simulink library "SUB_L4_Task_10ms_SUB_BRKPEDARB"  (R2018a)
settings: Solver=VariableStepAuto  StartTime=0.0  StopTime=10.0  RelTol=1e-3
libraries: EmE_MBD_Blockset x73, PTC_MBDS_LIB x6, simulink x3
(part 1 of 2)
settings Model: Creator=Chris.Balton  LastModifiedBy=Gavin.Coelho

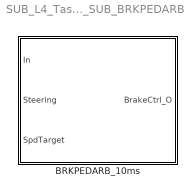
== system SUB_L4_Task_10ms_SUB_BRKPEDARB ==
  BRKPEDARB_10ms : Subsystem

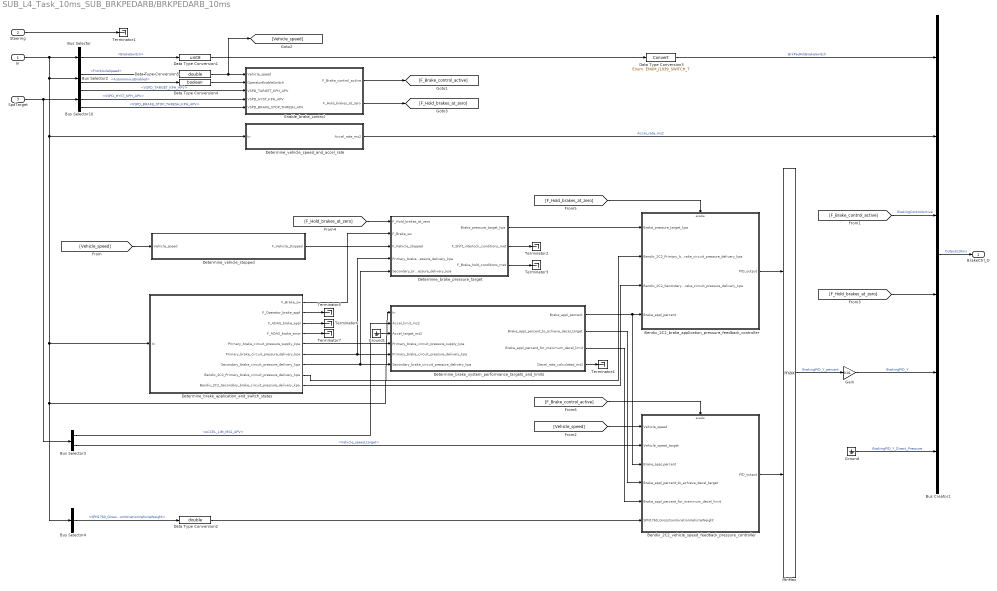
== system SUB_L4_Task_10ms_SUB_BRKPEDARB/BRKPEDARB_10ms ==
  In : Inport
  Steering : Inport  Port=2
  SpdTarget : Inport  Port=3
  Bendix_2C2_brake_application_pressure_feedback_controller : Subsystem  TreatAsAtomicUnit=on
  Bendix_2C2_vehicle_speed_feedback_pressure_controller : Subsystem  TreatAsAtomicUnit=on
  Bus Creator1 : BusCreator  Inputs=6
  Bus Selector : BusSelector  OutputSignals=CAN.CCVS_31.BrakeSwitch
  Bus Selector10 : BusSelector  OutputSignals=VSPD_TARGET_KPH_APV,VSPD_HYST_KPH_APV,VSPD_BRAKE_STOP_THRESH_KPH_APV
  Bus Selector2 : BusSelector  OutputSignals=CAN.EBC2_0B.FrontAxleSpeed,AutonomousState.AutonomousEnabled
  Bus Selector3 : BusSelector  OutputSignals=ACCEL_LIM_MS2_APV,Vehicle_speed_target
  Bus Selector4 : BusSelector  OutputSignals=CAN.CVW_0B.SPN1760_GrossCombinationVehicleWeight
  Data Type Conversion1 : DataTypeConversion  OutDataTypeStr=uint8  SaturateOnIntegerOverflow=on
  Data Type Conversion2 : DataTypeConversion  OutDataTypeStr=double  SaturateOnIntegerOverflow=on
  Data Type Conversion4 : DataTypeConversion  OutDataTypeStr=boolean  SaturateOnIntegerOverflow=on
  Data Type Conversion5 : DataTypeConversion  OutDataTypeStr=double  SaturateOnIntegerOverflow=on
  Data Type Conversion3 : DataTypeConversion  OutDataTypeStr=Enum: ENUM_J1939_SWITCH_T
      settings: AttributesFormatString=%<OutDataTypeStr>
  Determine_brake_application_and_switch_states : Subsystem
  Determine_brake_pressure_target : Subsystem
  Determine_brake_system_performance_targets_and_limits : Subsystem
  Determine_vehicle_speed_and_accel_rate : Subsystem
  Determine_vehicle_stopped : Subsystem
  Enable_brake_control : Subsystem
  Gain : Gain  Gain=0.01
  Ground : Ground
  Ground1 : Ground
  MinMax : MinMax  Function=max  Inputs=2  InputSameDT=on
  Terminator{1..7} (7 alike) : Terminator
      Terminator1 settings: InitFcn=|
      | try
      |    MBDS_BlockCallback('Update', gcb);
      | end
  BrakeCtrl_O : Outport
  wires:
  Bendix_2C2_vehicle_speed_feedback_pressure_controller/1(PID_output) -> MinMax/2
  Bendix_2C2_brake_application_pressure_feedback_controller/1(PID_output) -> MinMax/1
  [Vehicle_speed] -> Bendix_2C2_vehicle_speed_feedback_pressure_controller/1(Vehicle_speed)
  [F_Hold_brakes_at_zero] -> Bendix_2C2_brake_application_pressure_feedback_controller/Enable
  [F_Hold_brakes_at_zero] -> Determine_brake_pressure_target/1(F_Hold_brakes_at_zero)
  Ground1/1 -> Determine_brake_system_performance_targets_and_limits/3(Accel_target_ms2)
  [F_Hold_brakes_at_zero] -> Bus Creator1/4
  [F_Brake_control_active] -> Bus Creator1/3  "BrakingControlActive"
  Enable_brake_control/1(F_Brake_control_active) -> [F_Brake_control_active]
  Enable_brake_control/2(F_Hold_brakes_at_zero) -> [F_Hold_brakes_at_zero]
  [F_Brake_control_active] -> Bendix_2C2_vehicle_speed_feedback_pressure_controller/Enable
  Determine_brake_application_and_switch_states/8(Bendix_2C2_Primary_brake_circuit_pressure_delivery_kpa) -> Bendix_2C2_brake_application_pressure_feedback_controller/2(Bendix_2C2_Primary_brake_circuit_pressure_delivery_kpa)
  Determine_brake_application_and_switch_states/9(Bendix_2C2_Secondary_brake_circuit_pressure_delivery_kpa) -> Bendix_2C2_brake_application_pressure_feedback_controller/3(Bendix_2C2_Secondary_brake_circuit_pressure_delivery_kpa)
  [Vehicle_speed] -> Determine_vehicle_stopped/1(Vehicle_speed)
  Determine_vehicle_stopped/1(F_Vehicle_stopped) -> Determine_brake_pressure_target/3(F_Vehicle_stopped)
  Determine_brake_application_and_switch_states/1(F_Brake_sw) -> Determine_brake_pressure_target/2(F_Brake_sw)
  Determine_brake_application_and_switch_states/7(Secondary_brake_circuit_pressure_delivery_kpa) -> Determine_brake_pressure_target/5(Secondary_brake_circuit_pressure_delivery_kpa), Determine_brake_system_performance_targets_and_limits/6(Secondary_brake_circuit_pressure_delivery_kpa)
  Determine_brake_application_and_switch_states/5(Primary_brake_circuit_pressure_supply_kpa) -> Determine_brake_system_performance_targets_and_limits/4(Primary_brake_circuit_pressure_supply_kpa)
  Determine_brake_application_and_switch_states/6(Primary_brake_circuit_pressure_delivery_kpa) -> Determine_brake_pressure_target/4(Primary_brake_circuit_pressure_delivery_kpa), Determine_brake_system_performance_targets_and_limits/5(Primary_brake_circuit_pressure_delivery_kpa)
  Determine_brake_application_and_switch_states/4(F_ADAS_brake_error) -> Terminator7/1
  Determine_brake_application_and_switch_states/3(F_ADAS_brake_appl) -> Terminator6/1
  Determine_brake_application_and_switch_states/2(F_Operator_brake_appl) -> Terminator5/1
  Determine_brake_system_performance_targets_and_limits/4(Decel_rate_calculated_ms2) -> Terminator4/1
  Determine_brake_system_performance_targets_and_limits/3(Brake_appl_percent_for_maximum_decel_limit) -> Bendix_2C2_vehicle_speed_feedback_pressure_controller/5(Brake_appl_percent_for_maximum_decel_limit)
  Determine_brake_system_performance_targets_and_limits/2(Brake_appl_percent_to_achieve_decel_target) -> Bendix_2C2_vehicle_speed_feedback_pressure_controller/4(Brake_appl_percent_to_achieve_decel_target)
  Determine_brake_system_performance_targets_and_limits/1(Brake_appl_percent) -> Bendix_2C2_vehicle_speed_feedback_pressure_controller/3(Brake_appl_percent), Bendix_2C2_brake_application_pressure_feedback_controller/4(Brake_appl_percent)
  Determine_brake_pressure_target/3(F_Brake_hold_conditions_met) -> Terminator3/1
  Determine_brake_pressure_target/2(F_Shift_interlock_conditions_met) -> Terminator2/1
  Determine_brake_pressure_target/1(Brake_pressure_target_kpa) -> Bendix_2C2_brake_application_pressure_feedback_controller/1(Brake_pressure_target_kpa)
  Data Type Conversion3/1 -> Bus Creator1/1  "BrkPedArbBrakeSwitch"
  Determine_vehicle_speed_and_accel_rate/1(Accel_rate_ms2) -> Bus Creator1/2  "Accel_rate_ms2"
  Data Type Conversion4/1 -> Enable_brake_control/2(OperatorEnableSwitch)
  Data Type Conversion5/1 -> [Vehicle_speed], Enable_brake_control/1(Vehicle_speed)
  Data Type Conversion2/1 -> Bendix_2C2_vehicle_speed_feedback_pressure_controller/6(SPN1760_GrossCombinationVehicleWeight)
  Bus Selector2/2 -> Data Type Conversion4/1  "<AutonomousEnabled>"
  Bus Selector3/1 -> Determine_brake_system_performance_targets_and_limits/2(Accel_limit_ms2)  "<ACCEL_LIM_MS2_APV>"
  Bus Selector4/1 -> Data Type Conversion2/1  "<SPN1760_GrossCombinationVehicleWeight>"
  Bus Selector3/2 -> Bendix_2C2_vehicle_speed_feedback_pressure_controller/2(Vehicle_speed_target)  "<Vehicle_speed_target>"
  Bus Selector10/3 -> Enable_brake_control/5(VSPD_BRAKE_STOP_THRESH_APV)  "<VSPD_BRAKE_STOP_THRESH_KPH_APV>"
  Bus Selector10/1 -> Enable_brake_control/3(VSPD_TARGET_KPH_APV)  "<VSPD_TARGET_KPH_APV>"
  Bus Selector10/2 -> Enable_brake_control/4(VSPD_HYST_KPH_APV)  "<VSPD_HYST_KPH_APV>"
  Bus Selector2/1 -> Data Type Conversion5/1  "<FrontAxleSpeed>"
  SpdTarget/1 -> Bus Selector10/1, Bus Selector3/1
  In/1 -> Bus Selector2/1, Determine_vehicle_speed_and_accel_rate/1(In), Determine_brake_application_and_switch_states/1(In), Bus Selector4/1, Determine_brake_system_performance_targets_and_limits/1(In), Bus Selector/1
  Bus Creator1/1 -> BrakeCtrl_O/1  "Outputs10ms"
  Gain/1 -> Bus Creator1/5  "BrakingPID_Y"
  Data Type Conversion1/1 -> Data Type Conversion3/1
  Steering/1 -> Terminator1/1
  Bus Selector/1 -> Data Type Conversion1/1  "<BrakeSwitch>"
  Ground/1 -> Bus Creator1/6  "BrakingPID_Y_Direct_Pressure"
  MinMax/1 -> Gain/1  "BrakingPID_Y_percent"

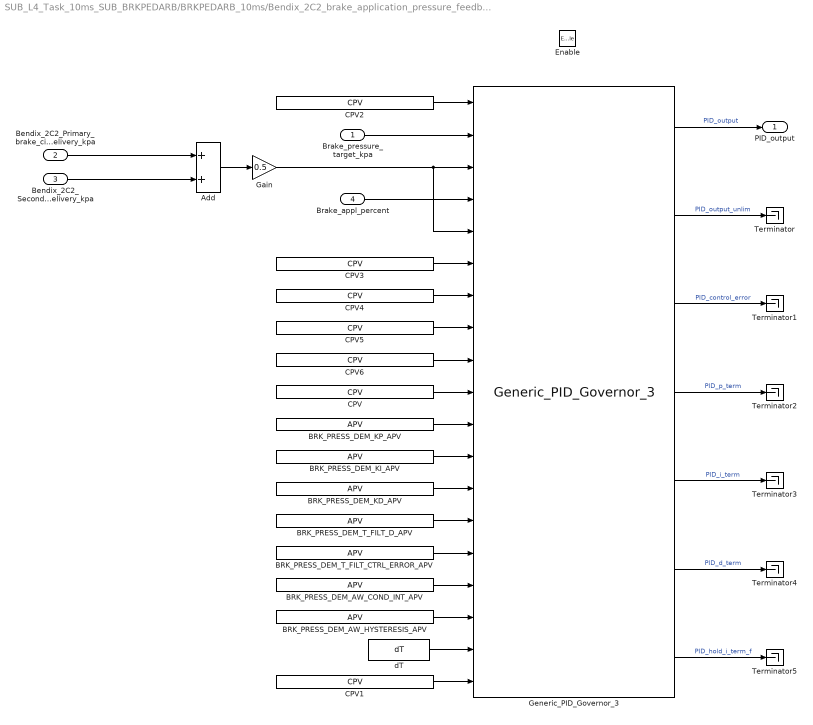
== system SUB_L4_Task_10ms_SUB_BRKPEDARB/BRKPEDARB_10ms/Bendix_2C2_brake_application_pressure_feedback_controller ==
  Brake_pressure_target_kpa : Inport
  Bendix_2C2_Primary_brake_circuit_pressure_delivery_kpa : Inport  Port=2
  Bendix_2C2_Secondary_brake_circuit_pressure_delivery_kpa : Inport  Port=3
  Brake_appl_percent : Inport  Port=4
  Enable : EnablePort  StatesWhenEnabling=reset
      settings: AttributesFormatString=States when enabling: %<StatesWhenEnabling>
      settings: CopyFcn=|
      | try
      | L = find_system(get(gcbh,'Parent'),'BlockType','Outport');
      | M = find_system(get(gcbh,'Parent'),'BlockType','EnablePort');
      | N = find_system(get(gcbh,'Parent'),'BlockType','TriggerPort');
      | anyoutports = ~isempty(L);
      | anyenableports = ~isempty(M);
      | anytriggerports = ~isempty(N);
      | sys = get_param(L,'Handle');
      | noutports = length(sys);
      | if (anyoutports),
      | for i = 1:noutports,
      | set(sys{i},'AttributesFormatString','IC: %<InitialOutput>\nDisabled value: %<OutputWhenDisabled>')
      | end;
      | end;
      | catch
      | end;
      | clear i L M N anyoutports anyenableports anytriggerports sys noutports
      settings: DeleteFcn=|
      | try
      | L = find_system(get(gcbh,'Parent'),'BlockType','Outport');
      | M = find_system(get(gcbh,'Parent'),'BlockType','EnablePort');
      | N = find_system(get(gcbh,'Parent'),'BlockType','TriggerPort');
      | anyoutports = ~isempty(L);
      | anyenableports = ~isempty(M);
      | anytriggerports = ~isempty(N);
      | sys = get_param(L,'Handle');
      | noutports = length(sys);
      | if ((anyoutports) && (~anytriggerports)),
      | for i = 1:noutports,
      | set(sys{i},'AttributesFormatString','')
      | end;
      | end;
      | catch
      | end;
      | clear i L M N anyoutports anyenableports anytriggerports sys noutports
      settings: NameChangeFcn=|
      | try
      | L = find_system(get(gcbh,'Parent'),'BlockType','Outport');
      | M = find_system(get(gcbh,'Parent'),'BlockType','EnablePort');
      | N = find_system(get(gcbh,'Parent'),'BlockType','TriggerPort');
      | anyoutports = ~isempty(L);
      | anyenableports = ~isempty(M);
      | anytriggerports = ~isempty(N);
      | sys = get_param(L,'Handle');
      | noutports = length(sys);
      | if (anyoutports),
      | for i = 1:noutports,
      | set(sys{i},'AttributesFormatString','IC: %<InitialOutput>\nDisabled value: %<OutputWhenDisabled>')
      | end;
      | end;
      | catch
      | end
      | clear i L M N anyoutports anyenableports anytriggerports sys noutports
      settings: MoveFcn=|
      | try
      | L = find_system(get(gcbh,'Parent'),'BlockType','Outport');
      | M = find_system(get(gcbh,'Parent'),'BlockType','EnablePort');
      | N = find_system(get(gcbh,'Parent'),'BlockType','TriggerPort');
      | anyoutports = ~isempty(L);
      | anyenableports = ~isempty(M);
      | anytriggerports = ~isempty(N);
      | sys = get_param(L,'Handle');
      | noutports = length(sys);
      | if (anyoutports),
      | for i = 1:noutports,
      | set(sys{i},'AttributesFormatString','IC: %<InitialOutput>\nDisabled value: %<OutputWhenDisabled>')
      | end;
      | end;
      | catch
      | end;
      | clear i L M N anyoutports anyenableports anytriggerports sys noutports
  Add : Sum  InputSameDT=on
  BRK_PRESS_DEM_AW_COND_INT_APV : EmE_MBD_Blockset/Sources/APV  conval=true
      settings: SourceProductName=PACCAR EmE MBD Blockset
  BRK_PRESS_DEM_AW_HYSTERESIS_APV : EmE_MBD_Blockset/Sources/APV  conval=7
      settings: SourceProductName=PACCAR EmE MBD Blockset
  BRK_PRESS_DEM_KD_APV : EmE_MBD_Blockset/Sources/APV  conval=0
      settings: SourceProductName=PACCAR EmE MBD Blockset
  BRK_PRESS_DEM_KI_APV : EmE_MBD_Blockset/Sources/APV  conval=0.1
      settings: SourceProductName=PACCAR EmE MBD Blockset
  BRK_PRESS_DEM_KP_APV : EmE_MBD_Blockset/Sources/APV  conval=0.05
      settings: SourceProductName=PACCAR EmE MBD Blockset
  BRK_PRESS_DEM_T_FILT_CTRL_ERROR_APV : EmE_MBD_Blockset/Sources/APV  conval=0.025
      settings: SourceProductName=PACCAR EmE MBD Blockset
  BRK_PRESS_DEM_T_FILT_D_APV : EmE_MBD_Blockset/Sources/APV  conval=0.025
      settings: SourceProductName=PACCAR EmE MBD Blockset
  CPV : EmE_MBD_Blockset/Sources/CPV  conval=0
      settings: SourceProductName=PACCAR EmE MBD Blockset
  CPV1 : EmE_MBD_Blockset/Sources/CPV  conval=false
      settings: SourceProductName=PACCAR EmE MBD Blockset
  CPV2 : EmE_MBD_Blockset/Sources/CPV  conval=false
      settings: SourceProductName=PACCAR EmE MBD Blockset
  CPV3 : EmE_MBD_Blockset/Sources/CPV  conval=0
      settings: SourceProductName=PACCAR EmE MBD Blockset
  CPV4 : EmE_MBD_Blockset/Sources/CPV  conval=5000
      settings: SourceProductName=PACCAR EmE MBD Blockset
  CPV5 : EmE_MBD_Blockset/Sources/CPV  conval=5000
      settings: SourceProductName=PACCAR EmE MBD Blockset
  CPV6 : EmE_MBD_Blockset/Sources/CPV  conval=100
      settings: SourceProductName=PACCAR EmE MBD Blockset
  Gain : Gain  Gain=0.5
  Generic_PID_Governor_3 : EmE_MBD_Blockset/Controllers/Generic_PID_Governor_3
      settings: SourceProductName=PACCAR EmE MBD Blockset
  Terminator{,1..5} (6 alike) : Terminator
  dT : EmE_MBD_Blockset/Sources/dT
      settings: SourceProductName=PACCAR EmE MBD Blockset
  PID_output : Outport  OutputWhenDisabled=reset  InitialOutput=0
      settings: AttributesFormatString=IC: %<InitialOutput>\nDisabled value: %<OutputWhenDisabled>
  wires:
  Gain/1 -> Generic_PID_Governor_3/3, Generic_PID_Governor_3/5
  Bendix_2C2_Secondary_brake_circuit_pressure_delivery_kpa/1 -> Add/2
  Bendix_2C2_Primary_brake_circuit_pressure_delivery_kpa/1 -> Add/1
  Add/1 -> Gain/1
  BRK_PRESS_DEM_KD_APV/1 -> Generic_PID_Governor_3/13
  BRK_PRESS_DEM_KI_APV/1 -> Generic_PID_Governor_3/12
  BRK_PRESS_DEM_KP_APV/1 -> Generic_PID_Governor_3/11
  CPV/1 -> Generic_PID_Governor_3/10
  Brake_pressure_target_kpa/1 -> Generic_PID_Governor_3/2
  CPV1/1 -> Generic_PID_Governor_3/19
  CPV4/1 -> Generic_PID_Governor_3/7
  CPV5/1 -> Generic_PID_Governor_3/8
  BRK_PRESS_DEM_T_FILT_D_APV/1 -> Generic_PID_Governor_3/14
  BRK_PRESS_DEM_T_FILT_CTRL_ERROR_APV/1 -> Generic_PID_Governor_3/15
  BRK_PRESS_DEM_AW_COND_INT_APV/1 -> Generic_PID_Governor_3/16
  BRK_PRESS_DEM_AW_HYSTERESIS_APV/1 -> Generic_PID_Governor_3/17
  dT/1 -> Generic_PID_Governor_3/18
  CPV2/1 -> Generic_PID_Governor_3/1
  Brake_appl_percent/1 -> Generic_PID_Governor_3/4
  CPV3/1 -> Generic_PID_Governor_3/6
  CPV6/1 -> Generic_PID_Governor_3/9
  Generic_PID_Governor_3/4 -> Terminator2/1  "PID_p_term"
  Generic_PID_Governor_3/3 -> Terminator1/1  "PID_control_error"
  Generic_PID_Governor_3/5 -> Terminator3/1  "PID_i_term"
  Generic_PID_Governor_3/2 -> Terminator/1  "PID_output_unlim"
  Generic_PID_Governor_3/6 -> Terminator4/1  "PID_d_term"
  Generic_PID_Governor_3/1 -> PID_output/1  "PID_output"
  Generic_PID_Governor_3/7 -> Terminator5/1  "PID_hold_i_term_f"

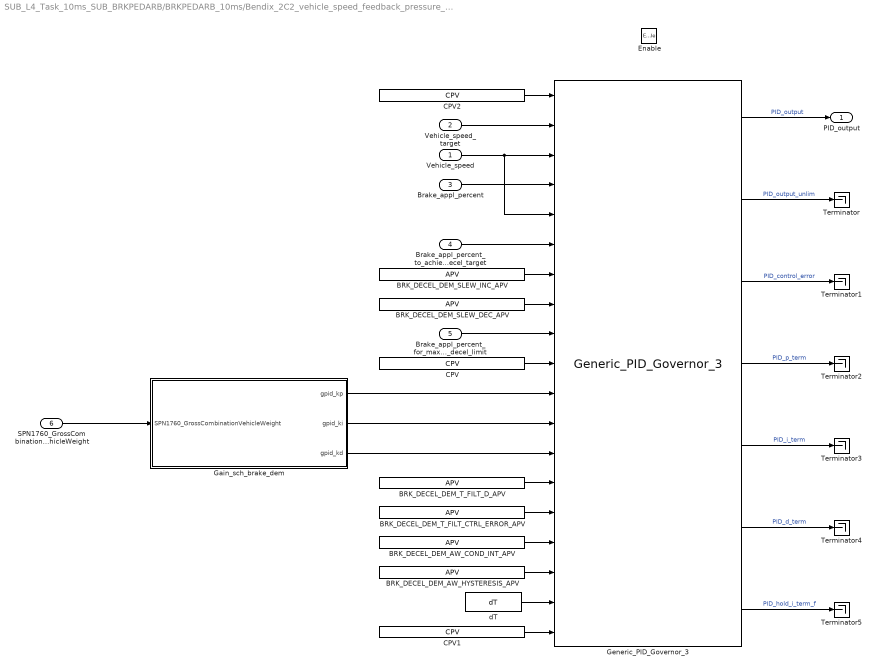
== system SUB_L4_Task_10ms_SUB_BRKPEDARB/BRKPEDARB_10ms/Bendix_2C2_vehicle_speed_feedback_pressure_controller ==
  Vehicle_speed : Inport
  Vehicle_speed_target : Inport  Port=2
  Brake_appl_percent : Inport  Port=3
  Brake_appl_percent_to_achieve_decel_target : Inport  Port=4
  Brake_appl_percent_for_maximum_decel_limit : Inport  Port=5
  SPN1760_GrossCombinationVehicleWeight : Inport  Port=6
  Enable : EnablePort  StatesWhenEnabling=reset
      settings: AttributesFormatString=States when enabling: %<StatesWhenEnabling>
      settings: CopyFcn=|
      | try
      | L = find_system(get(gcbh,'Parent'),'BlockType','Outport');
      | M = find_system(get(gcbh,'Parent'),'BlockType','EnablePort');
      | N = find_system(get(gcbh,'Parent'),'BlockType','TriggerPort');
      | anyoutports = ~isempty(L);
      | anyenableports = ~isempty(M);
      | anytriggerports = ~isempty(N);
      | sys = get_param(L,'Handle');
      | noutports = length(sys);
      | if (anyoutports),
      | for i = 1:noutports,
      | set(sys{i},'AttributesFormatString','IC: %<InitialOutput>\nDisabled value: %<OutputWhenDisabled>')
      | end;
      | end;
      | catch
      | end;
      | clear i L M N anyoutports anyenableports anytriggerports sys noutports
      settings: DeleteFcn=|
      | try
      | L = find_system(get(gcbh,'Parent'),'BlockType','Outport');
      | M = find_system(get(gcbh,'Parent'),'BlockType','EnablePort');
      | N = find_system(get(gcbh,'Parent'),'BlockType','TriggerPort');
      | anyoutports = ~isempty(L);
      | anyenableports = ~isempty(M);
      | anytriggerports = ~isempty(N);
      | sys = get_param(L,'Handle');
      | noutports = length(sys);
      | if ((anyoutports) && (~anytriggerports)),
      | for i = 1:noutports,
      | set(sys{i},'AttributesFormatString','')
      | end;
      | end;
      | catch
      | end;
      | clear i L M N anyoutports anyenableports anytriggerports sys noutports
      settings: NameChangeFcn=|
      | try
      | L = find_system(get(gcbh,'Parent'),'BlockType','Outport');
      | M = find_system(get(gcbh,'Parent'),'BlockType','EnablePort');
      | N = find_system(get(gcbh,'Parent'),'BlockType','TriggerPort');
      | anyoutports = ~isempty(L);
      | anyenableports = ~isempty(M);
      | anytriggerports = ~isempty(N);
      | sys = get_param(L,'Handle');
      | noutports = length(sys);
      | if (anyoutports),
      | for i = 1:noutports,
      | set(sys{i},'AttributesFormatString','IC: %<InitialOutput>\nDisabled value: %<OutputWhenDisabled>')
      | end;
      | end;
      | catch
      | end
      | clear i L M N anyoutports anyenableports anytriggerports sys noutports
      settings: MoveFcn=|
      | try
      | L = find_system(get(gcbh,'Parent'),'BlockType','Outport');
      | M = find_system(get(gcbh,'Parent'),'BlockType','EnablePort');
      | N = find_system(get(gcbh,'Parent'),'BlockType','TriggerPort');
      | anyoutports = ~isempty(L);
      | anyenableports = ~isempty(M);
      | anytriggerports = ~isempty(N);
      | sys = get_param(L,'Handle');
      | noutports = length(sys);
      | if (anyoutports),
      | for i = 1:noutports,
      | set(sys{i},'AttributesFormatString','IC: %<InitialOutput>\nDisabled value: %<OutputWhenDisabled>')
      | end;
      | end;
      | catch
      | end;
      | clear i L M N anyoutports anyenableports anytriggerports sys noutports
  BRK_DECEL_DEM_AW_COND_INT_APV : EmE_MBD_Blockset/Sources/APV  conval=true
      settings: SourceProductName=PACCAR EmE MBD Blockset
  BRK_DECEL_DEM_AW_HYSTERESIS_APV : EmE_MBD_Blockset/Sources/APV  conval=12
      settings: SourceProductName=PACCAR EmE MBD Blockset
  BRK_DECEL_DEM_SLEW_DEC_APV : EmE_MBD_Blockset/Sources/APV  conval=20
      settings: SourceProductName=PACCAR EmE MBD Blockset
  BRK_DECEL_DEM_SLEW_INC_APV : EmE_MBD_Blockset/Sources/APV  conval=20
      settings: SourceProductName=PACCAR EmE MBD Blockset
  BRK_DECEL_DEM_T_FILT_CTRL_ERROR_APV : EmE_MBD_Blockset/Sources/APV  conval=0.025
      settings: SourceProductName=PACCAR EmE MBD Blockset
  BRK_DECEL_DEM_T_FILT_D_APV : EmE_MBD_Blockset/Sources/APV  conval=0.4
      settings: SourceProductName=PACCAR EmE MBD Blockset
  CPV : EmE_MBD_Blockset/Sources/CPV  conval=0
      settings: SourceProductName=PACCAR EmE MBD Blockset
  CPV1 : EmE_MBD_Blockset/Sources/CPV  conval=false
      settings: SourceProductName=PACCAR EmE MBD Blockset
  CPV2 : EmE_MBD_Blockset/Sources/CPV  conval=false
      settings: SourceProductName=PACCAR EmE MBD Blockset
  Gain_sch_brake_dem : Subsystem
  Generic_PID_Governor_3 : EmE_MBD_Blockset/Controllers/Generic_PID_Governor_3
      settings: SourceProductName=PACCAR EmE MBD Blockset
  Terminator{,1..5} (6 alike) : Terminator
  dT : EmE_MBD_Blockset/Sources/dT
      settings: SourceProductName=PACCAR EmE MBD Blockset
  PID_output : Outport  OutputWhenDisabled=reset  InitialOutput=0
      settings: AttributesFormatString=IC: %<InitialOutput>\nDisabled value: %<OutputWhenDisabled>
  wires:
  Generic_PID_Governor_3/7 -> Terminator5/1  "PID_hold_i_term_f"
  Generic_PID_Governor_3/1 -> PID_output/1  "PID_output"
  Generic_PID_Governor_3/6 -> Terminator4/1  "PID_d_term"
  Generic_PID_Governor_3/2 -> Terminator/1  "PID_output_unlim"
  Generic_PID_Governor_3/5 -> Terminator3/1  "PID_i_term"
  Generic_PID_Governor_3/3 -> Terminator1/1  "PID_control_error"
  Generic_PID_Governor_3/4 -> Terminator2/1  "PID_p_term"
  Brake_appl_percent_for_maximum_decel_limit/1 -> Generic_PID_Governor_3/9
  Brake_appl_percent_to_achieve_decel_target/1 -> Generic_PID_Governor_3/6
  Brake_appl_percent/1 -> Generic_PID_Governor_3/4
  SPN1760_GrossCombinationVehicleWeight/1 -> Gain_sch_brake_dem/1(SPN1760_GrossCombinationVehicleWeight)
  CPV2/1 -> Generic_PID_Governor_3/1
  dT/1 -> Generic_PID_Governor_3/18
  BRK_DECEL_DEM_AW_HYSTERESIS_APV/1 -> Generic_PID_Governor_3/17
  BRK_DECEL_DEM_AW_COND_INT_APV/1 -> Generic_PID_Governor_3/16
  BRK_DECEL_DEM_T_FILT_CTRL_ERROR_APV/1 -> Generic_PID_Governor_3/15
  BRK_DECEL_DEM_T_FILT_D_APV/1 -> Generic_PID_Governor_3/14
  BRK_DECEL_DEM_SLEW_DEC_APV/1 -> Generic_PID_Governor_3/8
  BRK_DECEL_DEM_SLEW_INC_APV/1 -> Generic_PID_Governor_3/7
  Gain_sch_brake_dem/3(gpid_kd) -> Generic_PID_Governor_3/13
  Gain_sch_brake_dem/2(gpid_ki) -> Generic_PID_Governor_3/12
  Gain_sch_brake_dem/1(gpid_kp) -> Generic_PID_Governor_3/11
  CPV1/1 -> Generic_PID_Governor_3/19
  Vehicle_speed_target/1 -> Generic_PID_Governor_3/2
  Vehicle_speed/1 -> Generic_PID_Governor_3/3, Generic_PID_Governor_3/5
  CPV/1 -> Generic_PID_Governor_3/10

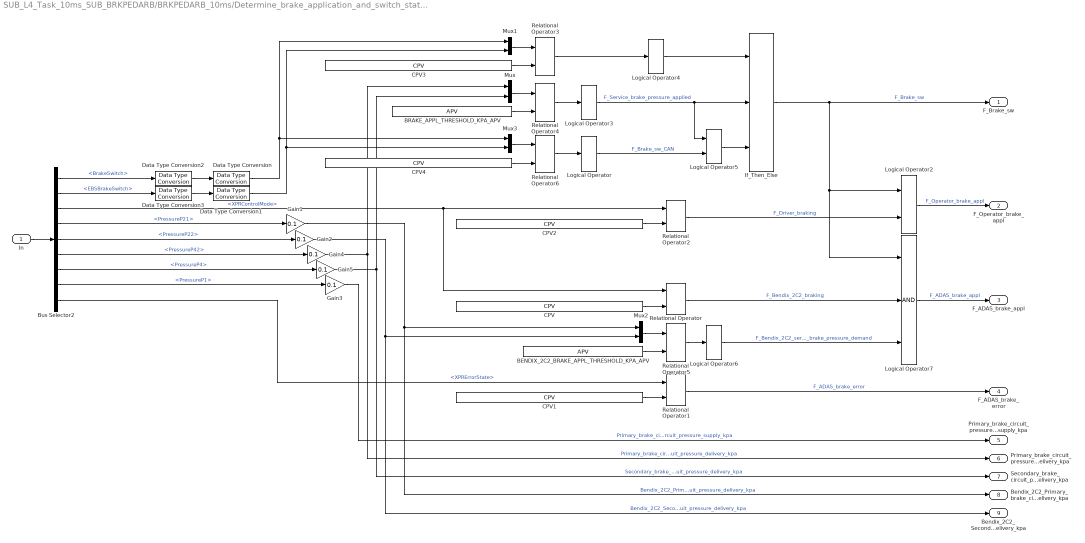
== system SUB_L4_Task_10ms_SUB_BRKPEDARB/BRKPEDARB_10ms/Determine_brake_application_and_switch_states ==
  In : Inport
  BENDIX_2C2_BRAKE_APPL_THRESHOLD_KPA_APV : EmE_MBD_Blockset/Sources/APV  conval=16
      settings: SourceProductName=PACCAR EmE MBD Blockset
  BRAKE_APPL_THRESHOLD_KPA_APV : EmE_MBD_Blockset/Sources/APV  conval=16
      settings: SourceProductName=PACCAR EmE MBD Blockset
  Bus Selector2 : BusSelector  OutputSignals=CAN.CCVS_31.BrakeSwitch,CAN.EBC1_0B.EBSBrakeSwitch,CAN.Prop2C2_Status_30.XPRControlMode,CAN.Prop2C2_Status_30.PressureP21,CAN.Prop2C2_Status_30.PressureP22,CAN.Prop2C2_Status_30.PressureP42,CAN.Prop2C2_Status_30.PressureP4,CAN.Prop2C2_Status_30.PressureP1,CAN.Prop2C2_Status_30.XPRErrorState
  CPV : EmE_MBD_Blockset/Sources/CPV  conval=ENUM_XPR_CONTROL_MODE_T.MAXIMUM_MODE
      settings: SourceProductName=PACCAR EmE MBD Blockset
  CPV1 : EmE_MBD_Blockset/Sources/CPV  conval=ENUM_XPR_ERROR_STATE_T.XPR_OK
      settings: SourceProductName=PACCAR EmE MBD Blockset
  CPV2 : EmE_MBD_Blockset/Sources/CPV  conval=ENUM_XPR_CONTROL_MODE_T.DRIVER_BRAKING_ONLY
      settings: SourceProductName=PACCAR EmE MBD Blockset
  CPV3 : EmE_MBD_Blockset/Sources/CPV  conval=ENUM_SWITCH_T.ERROR
      settings: SourceProductName=PACCAR EmE MBD Blockset
  CPV4 : EmE_MBD_Blockset/Sources/CPV  conval=ENUM_SWITCH_T.ON
      settings: SourceProductName=PACCAR EmE MBD Blockset
  Data Type Conversion : EmE_MBD_Blockset/Signal Attributes/Data Type Conversion  OutDataTypeStr=Enum: ENUM_SWITCH_T
      settings: AttributesFormatString=%<OutDataTypeStr>  SourceProductName=PACCAR EmE MBD Blockset
  Data Type Conversion1 : EmE_MBD_Blockset/Signal Attributes/Data Type Conversion  OutDataTypeStr=Enum: ENUM_SWITCH_T
      settings: AttributesFormatString=%<OutDataTypeStr>  SourceProductName=PACCAR EmE MBD Blockset
  Data Type Conversion2 : EmE_MBD_Blockset/Signal Attributes/Data Type Conversion  OutDataTypeStr=uint8
      settings: SourceProductName=PACCAR EmE MBD Blockset
  Data Type Conversion3 : EmE_MBD_Blockset/Signal Attributes/Data Type Conversion  OutDataTypeStr=uint8
      settings: SourceProductName=PACCAR EmE MBD Blockset
  Gain{1..5} (5 alike) : Gain  Gain=0.1
  If_Then_Else : EmE_MBD_Blockset/Signal Routing/If_Then_Else
      settings: SourceProductName=PACCAR EmE MBD Blockset
  Logical Operator : EmE_MBD_Blockset/Logic and Bit Operations/Logical Operator  Operator=OR  Inputs=1
      settings: SourceProductName=PACCAR EmE MBD Blockset
  Logical Operator2 : EmE_MBD_Blockset/Logic and Bit Operations/Logical Operator  Operator=AND  Inputs=2
      settings: SourceProductName=PACCAR EmE MBD Blockset
  Logical Operator3 : EmE_MBD_Blockset/Logic and Bit Operations/Logical Operator  Operator=OR  Inputs=1
      settings: SourceProductName=PACCAR EmE MBD Blockset
  Logical Operator4 : EmE_MBD_Blockset/Logic and Bit Operations/Logical Operator  Operator=AND  Inputs=1
      settings: SourceProductName=PACCAR EmE MBD Blockset
  Logical Operator5 : EmE_MBD_Blockset/Logic and Bit Operations/Logical Operator  Operator=OR  Inputs=2
      settings: SourceProductName=PACCAR EmE MBD Blockset
  Logical Operator6 : EmE_MBD_Blockset/Logic and Bit Operations/Logical Operator  Operator=OR  Inputs=1
      settings: SourceProductName=PACCAR EmE MBD Blockset
  Logical Operator7 : Logic  Inputs=3  OutDataTypeStr=boolean
  Mux{,1..3} (4 alike) : Mux  Inputs=2
  Relational Operator{,2..3,6} (4 alike) : EmE_MBD_Blockset/Logic and Bit Operations/Relational Operator  func===
      settings: SourceProductName=PACCAR EmE MBD Blockset
  Relational Operator1 : EmE_MBD_Blockset/Logic and Bit Operations/Relational Operator  func=~=
      settings: SourceProductName=PACCAR EmE MBD Blockset
  Relational Operator4 : EmE_MBD_Blockset/Logic and Bit Operations/Relational Operator  func=>
      settings: SourceProductName=PACCAR EmE MBD Blockset
  Relational Operator5 : EmE_MBD_Blockset/Logic and Bit Operations/Relational Operator  func=>
      settings: SourceProductName=PACCAR EmE MBD Blockset
  F_Brake_sw : Outport
  F_Operator_brake_appl : Outport  Port=2
  F_ADAS_brake_appl : Outport  Port=3
  F_ADAS_brake_error : Outport  Port=4
  Primary_brake_circuit_pressure_supply_kpa : Outport  Port=5
  Primary_brake_circuit_pressure_delivery_kpa : Outport  Port=6
  Secondary_brake_circuit_pressure_delivery_kpa : Outport  Port=7
  Bendix_2C2_Primary_brake_circuit_pressure_delivery_kpa : Outport  Port=8
  Bendix_2C2_Secondary_brake_circuit_pressure_delivery_kpa : Outport  Port=9
  wires:
  Data Type Conversion3/1 -> Data Type Conversion1/1
  Data Type Conversion2/1 -> Data Type Conversion/1
  Data Type Conversion1/1 -> Mux3/2, Mux1/2
  Data Type Conversion/1 -> Mux3/1, Mux1/1
  Logical Operator5/1 -> If_Then_Else/3
  Logical Operator6/1 -> Logical Operator7/3  "F_Bendix_2C2_service_brake_pressure_demand"
  Gain3/1 -> Primary_brake_circuit_pressure_supply_kpa/1  "Primary_brake_circuit_pressure_supply_kpa"
  Bus Selector2/8 -> Gain3/1  "<PressureP1>"
  Relational Operator6/1 -> Logical Operator/1
  CPV4/1 -> Relational Operator6/2
  Mux3/1 -> Relational Operator6/1
  Relational Operator5/1 -> Logical Operator6/1
  BENDIX_2C2_BRAKE_APPL_THRESHOLD_KPA_APV/1 -> Relational Operator5/2
  Gain2/1 -> Mux2/2, Bendix_2C2_Secondary_brake_circuit_pressure_delivery_kpa/1  "Bendix_2C2_Secondary_brake_circuit_pressure_delivery_kpa"
  Gain1/1 -> Mux2/1, Bendix_2C2_Primary_brake_circuit_pressure_delivery_kpa/1  "Bendix_2C2_Primary_brake_circuit_pressure_delivery_kpa"
  Mux2/1 -> Relational Operator5/1
  Bus Selector2/7 -> Gain5/1  "<PressureP4>"
  Bus Selector2/6 -> Gain4/1  "<PressureP42>"
  Bus Selector2/5 -> Gain2/1  "<PressureP22>"
  Gain5/1 -> Mux/2, Secondary_brake_circuit_pressure_delivery_kpa/1  "Secondary_brake_circuit_pressure_delivery_kpa"
  Gain4/1 -> Primary_brake_circuit_pressure_delivery_kpa/1, Mux/1  "Primary_brake_circuit_pressure_delivery_kpa"
  Logical Operator/1 -> Logical Operator5/2  "F_Brake_sw_CAN"
  Logical Operator4/1 -> If_Then_Else/1
  Mux1/1 -> Relational Operator3/1
  Bus Selector2/4 -> Gain1/1  "<PressureP21>"
  Mux/1 -> Relational Operator4/1
  Logical Operator3/1 -> If_Then_Else/2, Logical Operator5/1  "F_Service_brake_pressure_applied"
  Relational Operator4/1 -> Logical Operator3/1
  BRAKE_APPL_THRESHOLD_KPA_APV/1 -> Relational Operator4/2
  Relational Operator3/1 -> Logical Operator4/1
  CPV3/1 -> Relational Operator3/2
  Relational Operator2/1 -> Logical Operator2/2  "F_Driver_braking"
  Bus Selector2/3 -> Relational Operator2/1, Relational Operator/1  "<XPRControlMode>"
  CPV2/1 -> Relational Operator2/2
  Relational Operator1/1 -> F_ADAS_brake_error/1  "F_ADAS_brake_error"
  CPV1/1 -> Relational Operator1/2
  Bus Selector2/9 -> Relational Operator1/1  "<XPRErrorState>"
  CPV/1 -> Relational Operator/2
  Relational Operator/1 -> Logical Operator7/2  "F_Bendix_2C2_braking"
  Logical Operator7/1 -> F_ADAS_brake_appl/1  "F_ADAS_brake_appl"
  Logical Operator2/1 -> F_Operator_brake_appl/1  "F_Operator_brake_appl"
  If_Then_Else/1 -> Logical Operator2/1, Logical Operator7/1, F_Brake_sw/1  "F_Brake_sw"
  Bus Selector2/2 -> Data Type Conversion3/1  "<EBSBrakeSwitch>"
  In/1 -> Bus Selector2/1
  Bus Selector2/1 -> Data Type Conversion2/1  "<BrakeSwitch>"

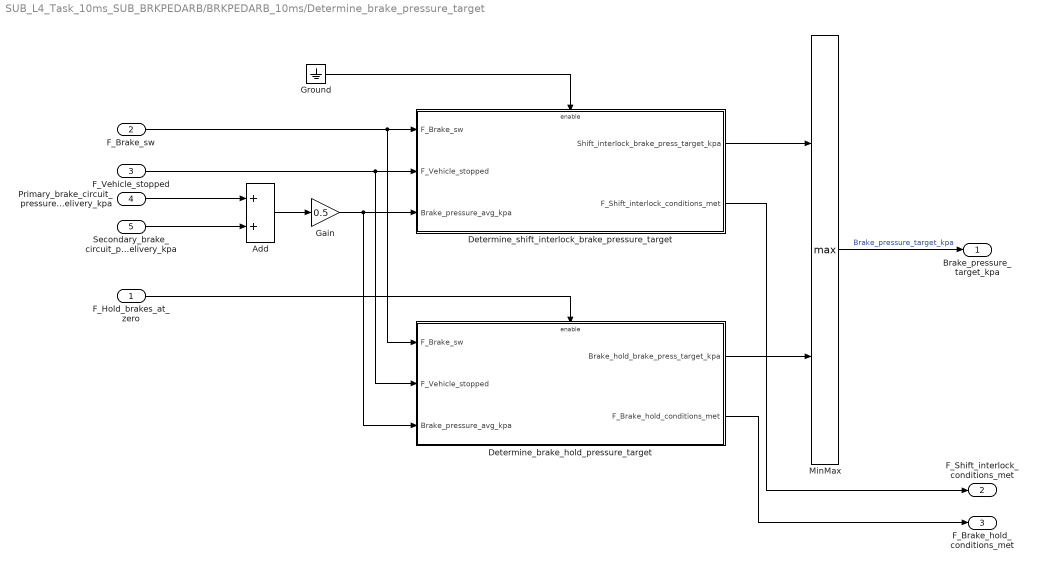
== system SUB_L4_Task_10ms_SUB_BRKPEDARB/BRKPEDARB_10ms/Determine_brake_pressure_target ==
  F_Hold_brakes_at_zero : Inport
  F_Brake_sw : Inport  Port=2
  F_Vehicle_stopped : Inport  Port=3
  Primary_brake_circuit_pressure_delivery_kpa : Inport  Port=4
  Secondary_brake_circuit_pressure_delivery_kpa : Inport  Port=5
  Add : Sum  InputSameDT=on
  Determine_brake_hold_pressure_target : Subsystem
  Determine_shift_interlock_brake_pressure_target : Subsystem
  Gain : Gain  Gain=0.5
  Ground : Ground
  MinMax : MinMax  Function=max  Inputs=2  InputSameDT=on
  Brake_pressure_target_kpa : Outport
  F_Shift_interlock_conditions_met : Outport  Port=2  OutputWhenDisabled=reset  InitialOutput=false
  F_Brake_hold_conditions_met : Outport  Port=3  OutputWhenDisabled=reset  InitialOutput=false
  wires:
  Ground/1 -> Determine_shift_interlock_brake_pressure_target/Enable
  Determine_brake_hold_pressure_target/2(F_Brake_hold_conditions_met) -> F_Brake_hold_conditions_met/1
  Determine_shift_interlock_brake_pressure_target/2(F_Shift_interlock_conditions_met) -> F_Shift_interlock_conditions_met/1
  F_Vehicle_stopped/1 -> Determine_shift_interlock_brake_pressure_target/2(F_Vehicle_stopped), Determine_brake_hold_pressure_target/2(F_Vehicle_stopped)
  F_Brake_sw/1 -> Determine_shift_interlock_brake_pressure_target/1(F_Brake_sw), Determine_brake_hold_pressure_target/1(F_Brake_sw)
  F_Hold_brakes_at_zero/1 -> Determine_brake_hold_pressure_target/Enable
  Determine_shift_interlock_brake_pressure_target/1(Shift_interlock_brake_press_target_kpa) -> MinMax/1
  Primary_brake_circuit_pressure_delivery_kpa/1 -> Add/1
  Secondary_brake_circuit_pressure_delivery_kpa/1 -> Add/2
  Add/1 -> Gain/1
  Gain/1 -> Determine_shift_interlock_brake_pressure_target/3(Brake_pressure_avg_kpa), Determine_brake_hold_pressure_target/3(Brake_pressure_avg_kpa)
  Determine_brake_hold_pressure_target/1(Brake_hold_brake_press_target_kpa) -> MinMax/2
  MinMax/1 -> Brake_pressure_target_kpa/1  "Brake_pressure_target_kpa"

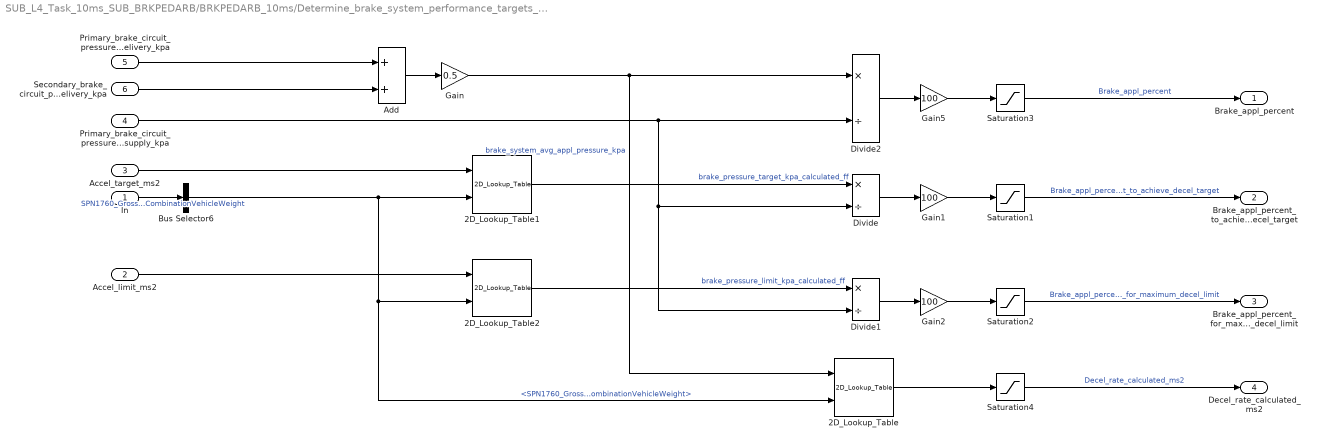
== system SUB_L4_Task_10ms_SUB_BRKPEDARB/BRKPEDARB_10ms/Determine_brake_system_performance_targets_and_limits ==
  In : Inport
  Accel_limit_ms2 : Inport  Port=2
  Accel_target_ms2 : Inport  Port=3
  Primary_brake_circuit_pressure_supply_kpa : Inport  Port=4
  Primary_brake_circuit_pressure_delivery_kpa : Inport  Port=5
  Secondary_brake_circuit_pressure_delivery_kpa : Inport  Port=6
  2D_Lookup_Table : PTC_MBDS_LIB/Extras/Lookup Tables/2D_Lookup_Table  ParameterObjectName=BRK_GOV_FF_DECEL_RATE_DATA_MPV  InterpolationMethod=Linear  PTC_MBDS_BlockVersion=5.41  PTC_BlockType=PTC_MBDS_2D_Lookup_Table
      settings: SourceProductName=PACCAR Technical Center MBDS Library
      settings: AttributesFormatString=|
      | Row Axis: BRK_GOV_FF_PRESS_KPA_STEP_MPV (kPa)
      | Column Axis: BRK_GOV_FF_MASS_STEP_MPV (kg)
      | Data Axis: BRK_GOV_FF_DECEL_RATE_DATA_MPV (m/s^2)
      | Interpolation Method: Linear
  2D_Lookup_Table1 : PTC_MBDS_LIB/Extras/Lookup Tables/2D_Lookup_Table  ParameterObjectName=BRK_GOV_FF_PRESS_KPA_DATA_MPV  InterpolationMethod=Linear  PTC_MBDS_BlockVersion=5.41  PTC_BlockType=PTC_MBDS_2D_Lookup_Table
      settings: SourceProductName=PACCAR Technical Center MBDS Library
      settings: AttributesFormatString=|
      | Row Axis: BRK_GOV_FF_DECEL_RATE_STEP_MPV (m/s^2)
      | Column Axis: BRK_GOV_FF_MASS_STEP_MPV (kg)
      | Data Axis: BRK_GOV_FF_PRESS_KPA_DATA_MPV (kPa)
      | Interpolation Method: Linear
  2D_Lookup_Table2 : PTC_MBDS_LIB/Extras/Lookup Tables/2D_Lookup_Table  ParameterObjectName=BRK_GOV_FF_PRESS_KPA_DATA_MPV  InterpolationMethod=Linear  PTC_MBDS_BlockVersion=5.41  PTC_BlockType=PTC_MBDS_2D_Lookup_Table
      settings: SourceProductName=PACCAR Technical Center MBDS Library
      settings: AttributesFormatString=|
      | Row Axis: BRK_GOV_FF_DECEL_RATE_STEP_MPV (m/s^2)
      | Column Axis: BRK_GOV_FF_MASS_STEP_MPV (kg)
      | Data Axis: BRK_GOV_FF_PRESS_KPA_DATA_MPV (kPa)
      | Interpolation Method: Linear
  Add : Sum  InputSameDT=on
  Bus Selector6 : BusSelector  OutputSignals=CAN.CVW_0B.SPN1760_GrossCombinationVehicleWeight
  Divide : Product  Inputs=*/  InputSameDT=on
  Divide1 : Product  Inputs=*/  InputSameDT=on
  Divide2 : Product  Inputs=*/  InputSameDT=on
  Gain : Gain  Gain=0.5
  Gain1 : Gain  Gain=100
  Gain2 : Gain  Gain=100
  Gain5 : Gain  Gain=100
  Saturation1 : Saturate  UpperLimit=100  LowerLimit=0
      settings: AttributesFormatString=|
      | Min: %<LowerLimit>
      | Max: %<UpperLimit>
  Saturation2 : Saturate  UpperLimit=100  LowerLimit=0
      settings: AttributesFormatString=|
      | Min: %<LowerLimit>
      | Max: %<UpperLimit>
  Saturation3 : Saturate  UpperLimit=100  LowerLimit=0
      settings: AttributesFormatString=|
      | Min: %<LowerLimit>
      | Max: %<UpperLimit>
  Saturation4 : Saturate  UpperLimit=0  LowerLimit=-15.687
      settings: AttributesFormatString=|
      | Min: %<LowerLimit>
      | Max: %<UpperLimit>
  Brake_appl_percent : Outport
  Brake_appl_percent_to_achieve_decel_target : Outport  Port=2
  Brake_appl_percent_for_maximum_decel_limit : Outport  Port=3
  Decel_rate_calculated_ms2 : Outport  Port=4
  wires:
  Saturation4/1 -> Decel_rate_calculated_ms2/1  "Decel_rate_calculated_ms2"
  Saturation3/1 -> Brake_appl_percent/1  "Brake_appl_percent"
  Saturation1/1 -> Brake_appl_percent_to_achieve_decel_target/1  "Brake_appl_percent_to_achieve_decel_target"
  Saturation2/1 -> Brake_appl_percent_for_maximum_decel_limit/1  "Brake_appl_percent_for_maximum_decel_limit"
  In/1 -> Bus Selector6/1  "SPN1760_GrossCombinationVehicleWeight"
  Accel_target_ms2/1 -> 2D_Lookup_Table1/1
  Divide2/1 -> Gain5/1
  Gain2/1 -> Saturation2/1
  2D_Lookup_Table/1 -> Saturation4/1
  Secondary_brake_circuit_pressure_delivery_kpa/1 -> Add/2
  2D_Lookup_Table1/1 -> Divide/1  "brake_pressure_target_kpa_calculated_ff"
  Gain5/1 -> Saturation3/1
  Accel_limit_ms2/1 -> 2D_Lookup_Table2/1
  Primary_brake_circuit_pressure_supply_kpa/1 -> Divide1/2, Divide/2, Divide2/2
  2D_Lookup_Table2/1 -> Divide1/1  "brake_pressure_limit_kpa_calculated_ff"
  Gain1/1 -> Saturation1/1
  Bus Selector6/1 -> 2D_Lookup_Table1/2, 2D_Lookup_Table2/2, 2D_Lookup_Table/2  "<SPN1760_GrossCombinationVehicleWeight>"
  Primary_brake_circuit_pressure_delivery_kpa/1 -> Add/1
  Gain/1 -> 2D_Lookup_Table/1, Divide2/1  "brake_system_avg_appl_pressure_kpa"
  Divide/1 -> Gain1/1
  Divide1/1 -> Gain2/1
  Add/1 -> Gain/1

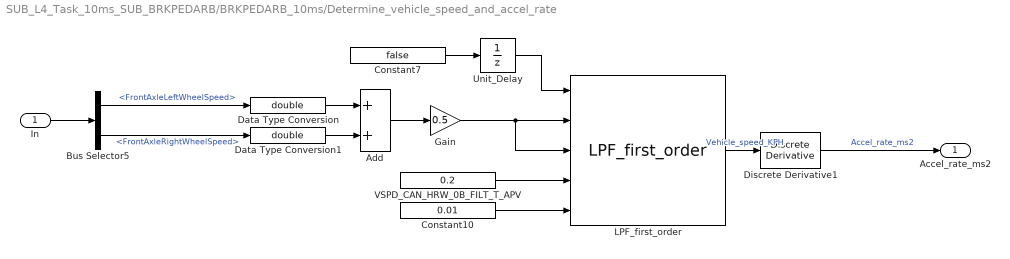
== system SUB_L4_Task_10ms_SUB_BRKPEDARB/BRKPEDARB_10ms/Determine_vehicle_speed_and_accel_rate ==
  In : Inport
  Add : Sum  InputSameDT=on
  Bus Selector5 : BusSelector  OutputSignals=CAN.HRW_0B.FrontAxleLeftWheelSpeed,CAN.HRW_0B.FrontAxleRightWheelSpeed
  Constant10 : Constant  Value=0.01
  Constant7 : Constant  Value=false
  Data Type Conversion : DataTypeConversion  OutDataTypeStr=double  SaturateOnIntegerOverflow=on
  Data Type Conversion1 : DataTypeConversion  OutDataTypeStr=double  SaturateOnIntegerOverflow=on
  Discrete Derivative1 : simulink/Discrete/Discrete Derivative  gainval=1.0  ICPrevScaledInput=0.0  InputProcessing=Inherited  OutMin=[]  OutMax=[]  OutDataTypeStr=double  OutputDataTypeScalingMode=double  OutDataType=fixdt(1, 16)  OutScaling=2^-10  DoSatur=off
  Gain : Gain  Gain=0.5  OutDataTypeStr=Inherit: Inherit via back propagation
  LPF_first_order : EmE_MBD_Blockset/Discrete/LPF_first_order
      settings: SourceProductName=PACCAR EmE MBD Blockset
  Unit_Delay : UnitDelay  InitialCondition=true  SampleTime=-1
      settings: AttributesFormatString=IC: %<vinit>
  VSPD_CAN_HRW_0B_FILT_T_APV : Constant  Value=0.2
  Accel_rate_ms2 : Outport
  wires:
  VSPD_CAN_HRW_0B_FILT_T_APV/1 -> LPF_first_order/4
  Discrete Derivative1/1 -> Accel_rate_ms2/1  "Accel_rate_ms2"
  Constant10/1 -> LPF_first_order/5
  Add/1 -> Gain/1
  Bus Selector5/2 -> Data Type Conversion1/1  "<FrontAxleRightWheelSpeed>"
  Bus Selector5/1 -> Data Type Conversion/1  "<FrontAxleLeftWheelSpeed>"
  Gain/1 -> LPF_first_order/2, LPF_first_order/3
  Constant7/1 -> Unit_Delay/1
  Unit_Delay/1 -> LPF_first_order/1
  LPF_first_order/1 -> Discrete Derivative1/1  "Vehicle_speed_KPH"
  In/1 -> Bus Selector5/1
  Data Type Conversion/1 -> Add/1
  Data Type Conversion1/1 -> Add/2

== system SUB_L4_Task_10ms_SUB_BRKPEDARB/BRKPEDARB_10ms/Determine_vehicle_stopped ==
  Vehicle_speed : Inport
  Relational Operator1 : EmE_MBD_Blockset/Logic and Bit Operations/Relational Operator  func=<=
      settings: SourceProductName=PACCAR EmE MBD Blockset
  SPN904_ZERO_SPD_CPV : EmE_MBD_Blockset/Sources/CPV  conval=0
      settings: SourceProductName=PACCAR EmE MBD Blockset
  F_Vehicle_stopped : Outport
  wires:
  SPN904_ZERO_SPD_CPV/1 -> Relational Operator1/2
  Vehicle_speed/1 -> Relational Operator1/1  "Vehicle_speed"
  Relational Operator1/1 -> F_Vehicle_stopped/1  "F_Vehicle_stopped"

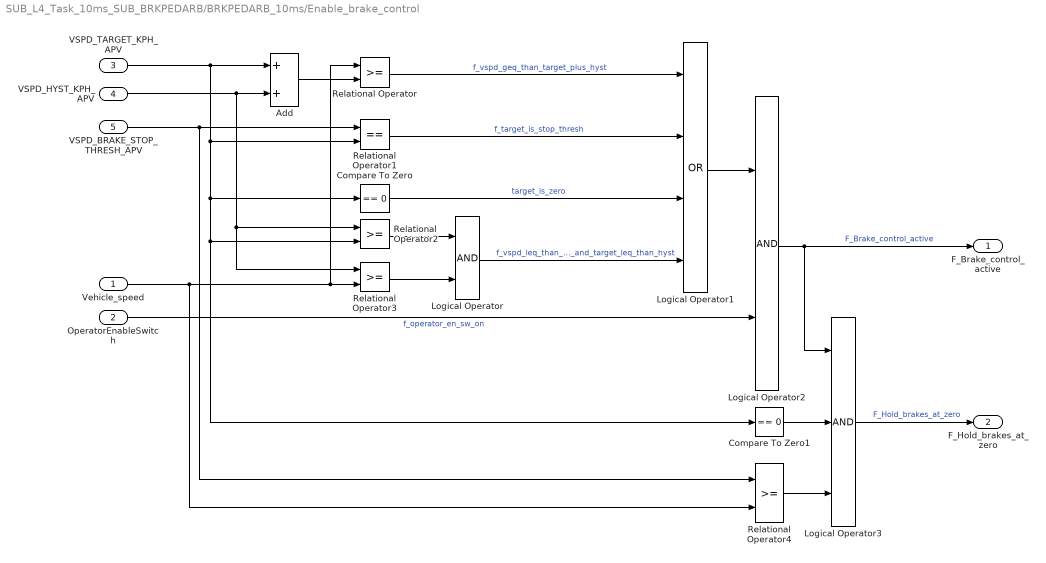
== system SUB_L4_Task_10ms_SUB_BRKPEDARB/BRKPEDARB_10ms/Enable_brake_control ==
  Vehicle_speed : Inport
  OperatorEnableSwitch : Inport  Port=2
  VSPD_TARGET_KPH_APV : Inport  Port=3
  VSPD_HYST_KPH_APV : Inport  Port=4
  VSPD_BRAKE_STOP_THRESH_APV : Inport  Port=5
  Add : Sum  InputSameDT=on
  Compare To Zero : simulink/Logic and Bit Operations/Compare To Zero  relop===  OutDataTypeStr=boolean
  Compare To Zero1 : simulink/Logic and Bit Operations/Compare To Zero  relop===  OutDataTypeStr=boolean
  Logical Operator : Logic  OutDataTypeStr=boolean
  Logical Operator1 : Logic  Operator=OR  Inputs=4  OutDataTypeStr=boolean
  Logical Operator2 : Logic  OutDataTypeStr=boolean
  Logical Operator3 : Logic  Inputs=3  AllPortsSameDT=off  OutDataTypeStr=boolean
  Relational Operator : RelationalOperator  OutDataTypeStr=boolean  RndMeth=Nearest  InputSameDT=on
  Relational Operator1 : RelationalOperator  Operator===  OutDataTypeStr=boolean  RndMeth=Nearest  InputSameDT=on
  Relational Operator2 : RelationalOperator  OutDataTypeStr=boolean  RndMeth=Nearest  InputSameDT=on
  Relational Operator3 : RelationalOperator  OutDataTypeStr=boolean  RndMeth=Nearest  InputSameDT=on
  Relational Operator4 : RelationalOperator  OutDataTypeStr=boolean  RndMeth=Nearest
  F_Brake_control_active : Outport
  F_Hold_brakes_at_zero : Outport  Port=2  OutputWhenDisabled=reset  InitialOutput=false
      settings: AttributesFormatString=IC: %<InitialOutput>\nDisabled value: %<OutputWhenDisabled>
  wires:
  Relational Operator4/1 -> Logical Operator3/3
  VSPD_TARGET_KPH_APV/1 -> Relational Operator2/2, Compare To Zero1/1, Compare To Zero/1, Relational Operator1/2, Add/1
  VSPD_BRAKE_STOP_THRESH_APV/1 -> Relational Operator1/1, Relational Operator4/1
  Logical Operator3/1 -> F_Hold_brakes_at_zero/1  "F_Hold_brakes_at_zero"
  Vehicle_speed/1 -> Relational Operator/1, Relational Operator3/2, Relational Operator4/2
  Compare To Zero1/1 -> Logical Operator3/2
  Logical Operator1/1 -> Logical Operator2/1
  OperatorEnableSwitch/1 -> Logical Operator2/2  "f_operator_en_sw_on"
  VSPD_HYST_KPH_APV/1 -> Add/2, Relational Operator2/1, Relational Operator3/1
  Add/1 -> Relational Operator/2
  Logical Operator2/1 -> F_Brake_control_active/1, Logical Operator3/1  "F_Brake_control_active"
  Relational Operator3/1 -> Logical Operator/2
  Relational Operator2/1 -> Logical Operator/1
  Logical Operator/1 -> Logical Operator1/4  "f_vspd_leq_than_hyst_and_target_leq_than_hyst"
  Compare To Zero/1 -> Logical Operator1/3  "target_is_zero"
  Relational Operator1/1 -> Logical Operator1/2  "f_target_is_stop_thresh"
  Relational Operator/1 -> Logical Operator1/1  "f_vspd_geq_than_target_plus_hyst"

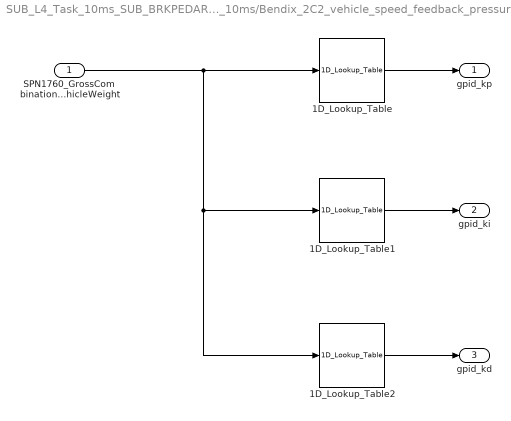
== system SUB_L4_Task_10ms_SUB_BRKPEDARB/BRKPEDARB_10ms/Bendix_2C2_vehicle_speed_feedback_pressure_controller/Gain_sch_brake_dem ==
  SPN1760_GrossCombinationVehicleWeight : Inport
  1D_Lookup_Table : PTC_MBDS_LIB/Extras/Lookup Tables/1D_Lookup_Table  ParameterObjectName=BRK_DEM_KP_DATA_MPV  InterpolationMethod=Linear  PTC_MBDS_BlockVersion=5.41  PTC_BlockType=PTC_MBDS_1D_Lookup_Table
      settings: SourceProductName=PACCAR Technical Center MBDS Library
      settings: AttributesFormatString=|
      | X Axis: BRK_DEM_MASS_STEP_MPV (kg)
      | Y Axis: BRK_DEM_KP_DATA_MPV (1)
      | Interpolation Method: Linear
  1D_Lookup_Table1 : PTC_MBDS_LIB/Extras/Lookup Tables/1D_Lookup_Table  ParameterObjectName=BRK_DEM_KI_DATA_MPV  InterpolationMethod=Linear  PTC_MBDS_BlockVersion=5.41  PTC_BlockType=PTC_MBDS_1D_Lookup_Table
      settings: SourceProductName=PACCAR Technical Center MBDS Library
      settings: AttributesFormatString=|
      | X Axis: BRK_DEM_MASS_STEP_MPV (kg)
      | Y Axis: BRK_DEM_KI_DATA_MPV (1/s)
      | Interpolation Method: Linear
  1D_Lookup_Table2 : PTC_MBDS_LIB/Extras/Lookup Tables/1D_Lookup_Table  ParameterObjectName=BRK_DEM_KD_DATA_MPV  InterpolationMethod=Linear  PTC_MBDS_BlockVersion=5.41  PTC_BlockType=PTC_MBDS_1D_Lookup_Table
      settings: SourceProductName=PACCAR Technical Center MBDS Library
      settings: AttributesFormatString=|
      | X Axis: BRK_DEM_MASS_STEP_MPV (kg)
      | Y Axis: BRK_DEM_KD_DATA_MPV (s)
      | Interpolation Method: Linear
  gpid_kp : Outport
  gpid_ki : Outport  Port=2
  gpid_kd : Outport  Port=3
  wires:
  1D_Lookup_Table2/1 -> gpid_kd/1
  1D_Lookup_Table1/1 -> gpid_ki/1
  SPN1760_GrossCombinationVehicleWeight/1 -> 1D_Lookup_Table/1, 1D_Lookup_Table2/1, 1D_Lookup_Table1/1
  1D_Lookup_Table/1 -> gpid_kp/1

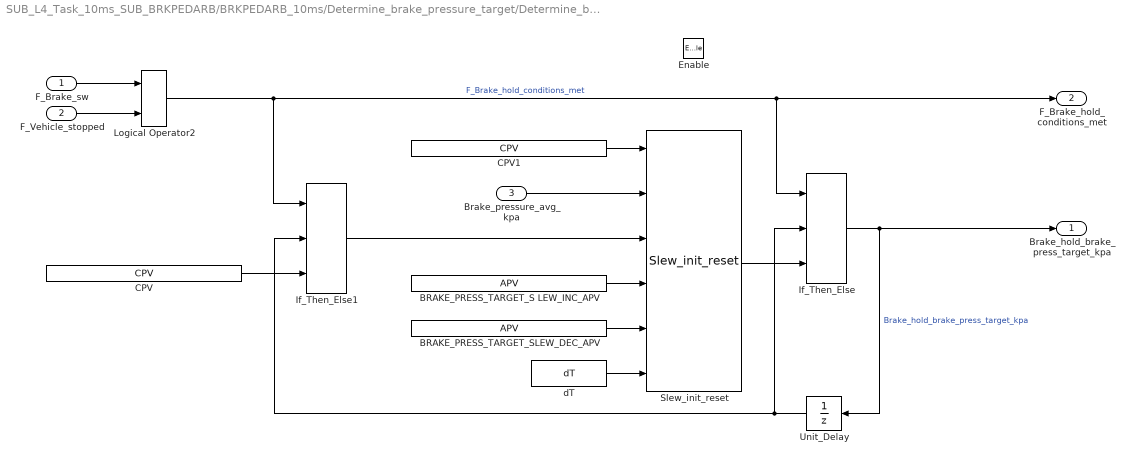
== system SUB_L4_Task_10ms_SUB_BRKPEDARB/BRKPEDARB_10ms/Determine_brake_pressure_target/Determine_brake_hold_pressure_target ==
  F_Brake_sw : Inport
  F_Vehicle_stopped : Inport  Port=2
  Brake_pressure_avg_kpa : Inport  Port=3
  Enable : EnablePort  StatesWhenEnabling=reset
      settings: AttributesFormatString=States when enabling: %<StatesWhenEnabling>
      settings: CopyFcn=|
      | try
      | L = find_system(get(gcbh,'Parent'),'BlockType','Outport');
      | M = find_system(get(gcbh,'Parent'),'BlockType','EnablePort');
      | N = find_system(get(gcbh,'Parent'),'BlockType','TriggerPort');
      | anyoutports = ~isempty(L);
      | anyenableports = ~isempty(M);
      | anytriggerports = ~isempty(N);
      | sys = get_param(L,'Handle');
      | noutports = length(sys);
      | if (anyoutports),
      | for i = 1:noutports,
      | set(sys{i},'AttributesFormatString','IC: %<InitialOutput>\nDisabled value: %<OutputWhenDisabled>')
      | end;
      | end;
      | catch
      | end;
      | clear i L M N anyoutports anyenableports anytriggerports sys noutports
      settings: DeleteFcn=|
      | try
      | L = find_system(get(gcbh,'Parent'),'BlockType','Outport');
      | M = find_system(get(gcbh,'Parent'),'BlockType','EnablePort');
      | N = find_system(get(gcbh,'Parent'),'BlockType','TriggerPort');
      | anyoutports = ~isempty(L);
      | anyenableports = ~isempty(M);
      | anytriggerports = ~isempty(N);
      | sys = get_param(L,'Handle');
      | noutports = length(sys);
      | if ((anyoutports) && (~anytriggerports)),
      | for i = 1:noutports,
      | set(sys{i},'AttributesFormatString','')
      | end;
      | end;
      | catch
      | end;
      | clear i L M N anyoutports anyenableports anytriggerports sys noutports
      settings: NameChangeFcn=|
      | try
      | L = find_system(get(gcbh,'Parent'),'BlockType','Outport');
      | M = find_system(get(gcbh,'Parent'),'BlockType','EnablePort');
      | N = find_system(get(gcbh,'Parent'),'BlockType','TriggerPort');
      | anyoutports = ~isempty(L);
      | anyenableports = ~isempty(M);
      | anytriggerports = ~isempty(N);
      | sys = get_param(L,'Handle');
      | noutports = length(sys);
      | if (anyoutports),
      | for i = 1:noutports,
      | set(sys{i},'AttributesFormatString','IC: %<InitialOutput>\nDisabled value: %<OutputWhenDisabled>')
      | end;
      | end;
      | catch
      | end
      | clear i L M N anyoutports anyenableports anytriggerports sys noutports
      settings: MoveFcn=|
      | try
      | L = find_system(get(gcbh,'Parent'),'BlockType','Outport');
      | M = find_system(get(gcbh,'Parent'),'BlockType','EnablePort');
      | N = find_system(get(gcbh,'Parent'),'BlockType','TriggerPort');
      | anyoutports = ~isempty(L);
      | anyenableports = ~isempty(M);
      | anytriggerports = ~isempty(N);
      | sys = get_param(L,'Handle');
      | noutports = length(sys);
      | if (anyoutports),
      | for i = 1:noutports,
      | set(sys{i},'AttributesFormatString','IC: %<InitialOutput>\nDisabled value: %<OutputWhenDisabled>')
      | end;
      | end;
      | catch
      | end;
      | clear i L M N anyoutports anyenableports anytriggerports sys noutports
  BRAKE_PRESS_TARGET_S LEW_INC_APV : EmE_MBD_Blockset/Sources/APV  conval=30
      settings: SourceProductName=PACCAR EmE MBD Blockset
  BRAKE_PRESS_TARGET_SLEW_DEC_APV : EmE_MBD_Blockset/Sources/APV  conval=5000
      settings: SourceProductName=PACCAR EmE MBD Blockset
  CPV : EmE_MBD_Blockset/Sources/CPV  conval=865
      settings: SourceProductName=PACCAR EmE MBD Blockset
  CPV1 : EmE_MBD_Blockset/Sources/CPV  conval=false
      settings: SourceProductName=PACCAR EmE MBD Blockset
  If_Then_Else : EmE_MBD_Blockset/Signal Routing/If_Then_Else
      settings: SourceProductName=PACCAR EmE MBD Blockset
  If_Then_Else1 : EmE_MBD_Blockset/Signal Routing/If_Then_Else
      settings: SourceProductName=PACCAR EmE MBD Blockset
  Logical Operator2 : EmE_MBD_Blockset/Logic and Bit Operations/Logical Operator  Operator=AND  Inputs=2
      settings: SourceProductName=PACCAR EmE MBD Blockset
  Slew_init_reset : EmE_MBD_Blockset/Math Operators/Slew_init_reset
      settings: SourceProductName=PACCAR EmE MBD Blockset
  Unit_Delay : UnitDelay  SampleTime=-1
      settings: AttributesFormatString=IC: %<vinit>
  dT : EmE_MBD_Blockset/Sources/dT
      settings: SourceProductName=PACCAR EmE MBD Blockset
  Brake_hold_brake_press_target_kpa : Outport  OutputWhenDisabled=reset  InitialOutput=0
      settings: AttributesFormatString=IC: %<InitialOutput>\nDisabled value: %<OutputWhenDisabled>
  F_Brake_hold_conditions_met : Outport  Port=2  OutputWhenDisabled=reset  InitialOutput=false
      settings: AttributesFormatString=IC: %<InitialOutput>\nDisabled value: %<OutputWhenDisabled>
  wires:
  CPV1/1 -> Slew_init_reset/1
  If_Then_Else1/1 -> Slew_init_reset/3
  F_Brake_sw/1 -> Logical Operator2/1
  F_Vehicle_stopped/1 -> Logical Operator2/2
  CPV/1 -> If_Then_Else1/3
  BRAKE_PRESS_TARGET_SLEW_DEC_APV/1 -> Slew_init_reset/5
  If_Then_Else/1 -> Unit_Delay/1, Brake_hold_brake_press_target_kpa/1  "Brake_hold_brake_press_target_kpa"
  Unit_Delay/1 -> If_Then_Else1/2, If_Then_Else/2
  Slew_init_reset/1 -> If_Then_Else/3
  dT/1 -> Slew_init_reset/6
  BRAKE_PRESS_TARGET_S LEW_INC_APV/1 -> Slew_init_reset/4
  Logical Operator2/1 -> If_Then_Else1/1, If_Then_Else/1, F_Brake_hold_conditions_met/1  "F_Brake_hold_conditions_met"
  Brake_pressure_avg_kpa/1 -> Slew_init_reset/2
